simulink model "Divide"  (R2015b)
settings: Solver=VariableStepAuto  StartTime=0.0  StopTime=10.0  RelTol=1e-3
settings Model: Creator=LUBO  LastModifiedBy=LUBO

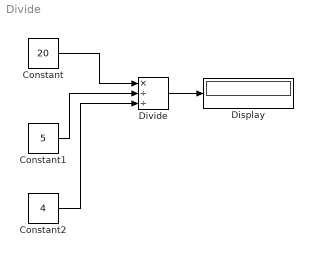
== system Divide ==
  Constant : Constant  Value=20
  Constant1 : Constant  Value=5
  Constant2 : Constant  Value=4
  Display : Display
  Divide : Product  Inputs=*//
  wires:
  Constant/1 -> Divide/1
  Constant2/1 -> Divide/3
  Constant1/1 -> Divide/2
  Divide/1 -> Display/1
